simulink model "pitch_control"  (R2020a)
settings: Solver=FixedStepAuto  StartTime=0.0  StopTime=10.0  FixedStep=step_size  RelTol=1e-3
values from neighbouring files (symbols this model uses):
  pitch_tf = tf([omega_n^2*pl], [1 2*zeta*omega_n omega_n^2])*tf([1],[1 pl],'InputDelay',0.09)    [untitled.m]
settings Model: Creator=pala  LastModifiedBy=pala
settings DataIOCC: SaveFormat=StructureWithTime

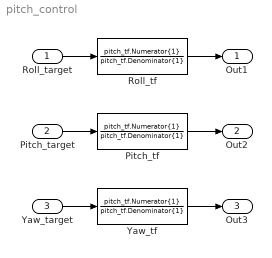
== system pitch_control ==
  Roll_target : Inport
  Pitch_target : Inport  Port=2
  Yaw_target : Inport  Port=3
  Pitch_tf : TransferFcn  Numerator=pitch_tf.Numerator{1}  Denominator=pitch_tf.Denominator{1}
  Roll_tf : TransferFcn  Numerator=pitch_tf.Numerator{1}  Denominator=pitch_tf.Denominator{1}
  Yaw_tf : TransferFcn  Numerator=pitch_tf.Numerator{1}  Denominator=pitch_tf.Denominator{1}
  Out1 : Outport
  Out2 : Outport  Port=2
  Out3 : Outport  Port=3
  wires:
  Roll_target/1 -> Roll_tf/1
  Roll_tf/1 -> Out1/1
  Pitch_tf/1 -> Out2/1
  Pitch_target/1 -> Pitch_tf/1
  Yaw_tf/1 -> Out3/1
  Yaw_target/1 -> Yaw_tf/1
